simulink model "cooperative_observer"  (R2024b)
settings: Solver=VariableStepAuto  StartTime=0.0  StopTime=200  RelTol=1e-3
values from neighbouring files (symbols this model uses):
  A0 = A-B*K0    [Project.m]    (also in analyze_Ag_components.m = A - B*K0; analyze_Ao_components.m = A - B*K0; debug_simulink_integration.m = A - B*K0; local_observer_design.m = A - B*K0)
  Adj = ones(N, N) - eye(N)    [create_network_topology.m]    (also in debug_simulink_integration.m = zeros(N))
  B = [0; -9.9453]    [Project.m]    (also in debug_simulink_integration.m; find_hurwitz_F.m = c * eye(n); project_multiple_run.m; project_single_run.m)
  C = [708.27 0]    [Project.m]    (also in debug_simulink_integration.m; project_multiple_run.m; project_single_run.m)
  c = cmin * 2    [Project.m]    (also in project_multiple_run.m = cmin * c_weights(ic); project_single_run.m = cmin)
  D = zeros(1,2)    [Project.m]    (also in debug_simulink_integration.m = zeros(size(C,1), size(B,2)); project_multiple_run.m = zeros(1, 2); project_single_run.m = zeros(1, 2))
  F = P * C' * R^(-1)    [Project.m]    (also in find_hurwitz_F.m = reshape(F_opt, n, p); local_observer_design.m = place(A0', C', desired_poles)')
  G = zeros(N, N)    [create_network_topology.m]    (also in debug_simulink_integration.m = zeros(N))
  K = R^(-1) * B' *Pc    [Project.m]    (also in find_hurwitz_F.m = lqr(A, B, Q, R); project_multiple_run.m = R^(-1) * B' * Pc; project_single_run.m = R^(-1) * B' * Pc)
  L0 = place(A', C', [-10, -20])'    [Project.m]    (also in project_multiple_run.m = place(A0', C', [-10, -20])'; project_single_run.m = place(A0', C', [-10, -20])')
  x0_0 = [Amp 0]'    [Project.m]    (also in project_multiple_run.m = [Amp; 0]; project_single_run.m = [Amp; 0]; setup_ramp_parameters.m = [initial_value; slope; 0])
  x0_1 = [0 0]'    [Project.m]    (also in project_multiple_run.m = perturb(x0_0); project_single_run.m = perturb(x0_0))
  x0_2 = [0 0]'    [Project.m]    (also in project_multiple_run.m = perturb(x0_0); project_single_run.m = perturb(x0_0))
  x0_3 = [0 0]'    [Project.m]    (also in project_multiple_run.m = perturb(x0_0); project_single_run.m = perturb(x0_0))
  x0_4 = [0 0]'    [Project.m]    (also in project_multiple_run.m = perturb(x0_0); project_single_run.m = perturb(x0_0))
  x0_5 = [0 0]'    [Project.m]    (also in project_multiple_run.m = perturb(x0_0); project_single_run.m = perturb(x0_0))
  x0_6 = [0 0]'    [Project.m]    (also in project_multiple_run.m = perturb(x0_0); project_single_run.m = perturb(x0_0))
settings Model: Creator=fvero  LastModifiedBy=Ing. Dario Lupo

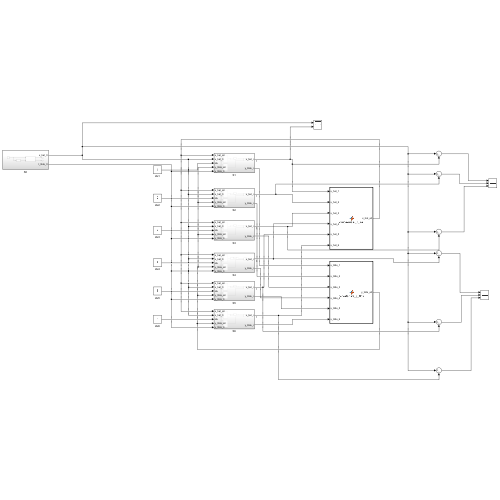
[thumbnail: Simulink's stored preview of the top-level diagram]
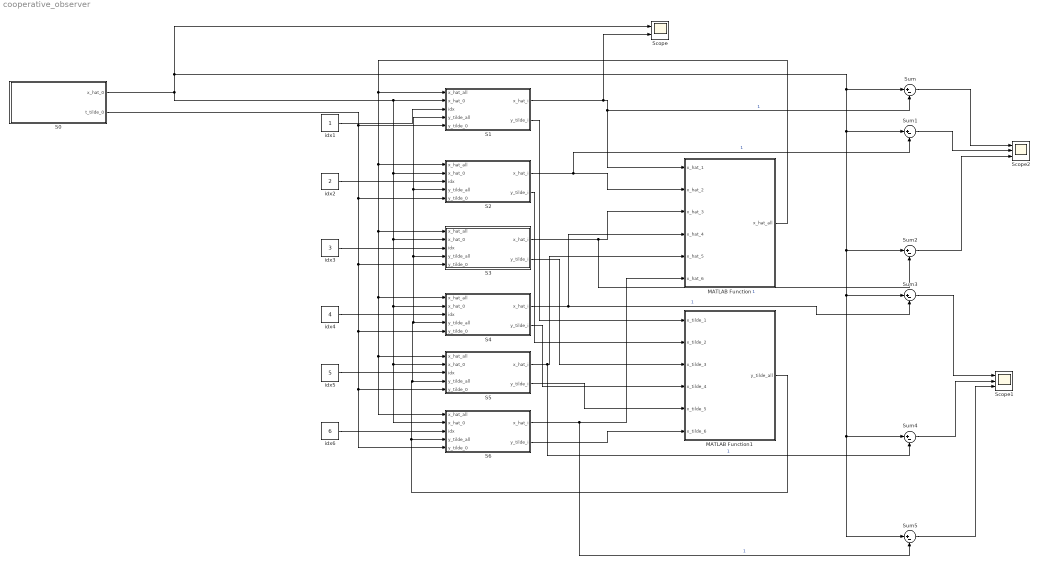
== system cooperative_observer ==
  MATLAB Function : MATLAB Function  TreatAsAtomicUnit=on
  MATLAB Function1 : MATLAB Function  TreatAsAtomicUnit=on
  S0 : Subsystem
  S1 : Subsystem
  S2 : Subsystem
  S3 : Subsystem
  S4 : Subsystem
  S5 : Subsystem
  S6 : Subsystem
  Scope : Scope  NumInputPorts=2
  Scope1 : Scope  NumInputPorts=3
  Scope2 : Scope  NumInputPorts=3
  Sum{,1..5} (6 alike) : Sum  Inputs=|+-
  idx1 : Constant
  idx2 : Constant  Value=2
  idx3 : Constant  Value=3
  idx4 : Constant  Value=4
  idx5 : Constant  Value=5
  idx6 : Constant  Value=6
  wires:
  MATLAB Function/1(x_hat_all) -> S6/1(x_hat_all), S5/1(x_hat_all), S4/1(x_hat_all), S3/1(x_hat_all), S2/1(x_hat_all), S1/1(x_hat_all)
  idx1/1 -> S1/3(idx)
  idx2/1 -> S2/3(idx)
  idx3/1 -> S3/3(idx)
  idx4/1 -> S4/3(idx)
  idx6/1 -> S6/3(idx)
  idx5/1 -> S5/3(idx)
  S0/1(x_hat_0) -> S6/2(x_hat_0), S5/2(x_hat_0), S4/2(x_hat_0), S3/2(x_hat_0), S2/2(x_hat_0), S1/2(x_hat_0), Scope/1, Sum4/1, Sum5/1, Sum3/1, Sum2/1, Sum1/1, Sum/1
  S1/1(x_hat_i) -> Scope/2, Sum/2, MATLAB Function/1(x_hat_1)  "1"
  S2/1(x_hat_i) -> Sum1/2, MATLAB Function/2(x_hat_2)  "1"
  S3/1(x_hat_i) -> Sum2/2, MATLAB Function/3(x_hat_3)  "1"
  S4/1(x_hat_i) -> Sum3/2, MATLAB Function/4(x_hat_4)  "1"
  S5/1(x_hat_i) -> Sum4/2, MATLAB Function/5(x_hat_5)  "1"
  S6/1(x_hat_i) -> Sum5/2, MATLAB Function/6(x_hat_6)  "1"
  S1/2(y_tilde_i) -> MATLAB Function1/1(x_tilde_1)
  S2/2(y_tilde_i) -> MATLAB Function1/2(x_tilde_2)
  S3/2(y_tilde_i) -> MATLAB Function1/3(x_tilde_3)
  S4/2(y_tilde_i) -> MATLAB Function1/4(x_tilde_4)
  S5/2(y_tilde_i) -> MATLAB Function1/5(x_tilde_5)
  S6/2(y_tilde_i) -> MATLAB Function1/6(x_tilde_6)
  MATLAB Function1/1(y_tilde_all) -> S2/4(y_tilde_all), S1/4(y_tilde_all), S3/4(y_tilde_all), S4/4(y_tilde_all), S5/4(y_tilde_all), S6/4(y_tilde_all)
  S0/2(t_tilde_0) -> S6/5(y_tilde_0), S5/5(y_tilde_0), S4/5(y_tilde_0), S3/5(y_tilde_0), S2/5(y_tilde_0), S1/5(y_tilde_0)
  Sum/1 -> Scope2/1
  Sum1/1 -> Scope2/2
  Sum2/1 -> Scope2/3
  Sum3/1 -> Scope1/1
  Sum4/1 -> Scope1/2
  Sum5/1 -> Scope1/3

== system cooperative_observer/S0 ==
  Constant : Constant  Value=0
  Leader Observer : Subsystem
  State-Space : StateSpace  A=A0  B=B  C=C  D=0  InitialCondition=x0_0
  x_hat_0 : Outport
  t_tilde_0 : Outport  Port=2
  wires:
  State-Space/1 -> Leader Observer/2(y)
  Constant/1 -> State-Space/1, Leader Observer/1(u)
  Leader Observer/1(x_hat_0) -> x_hat_0/1
  Leader Observer/2(t_tilde_0) -> t_tilde_0/1

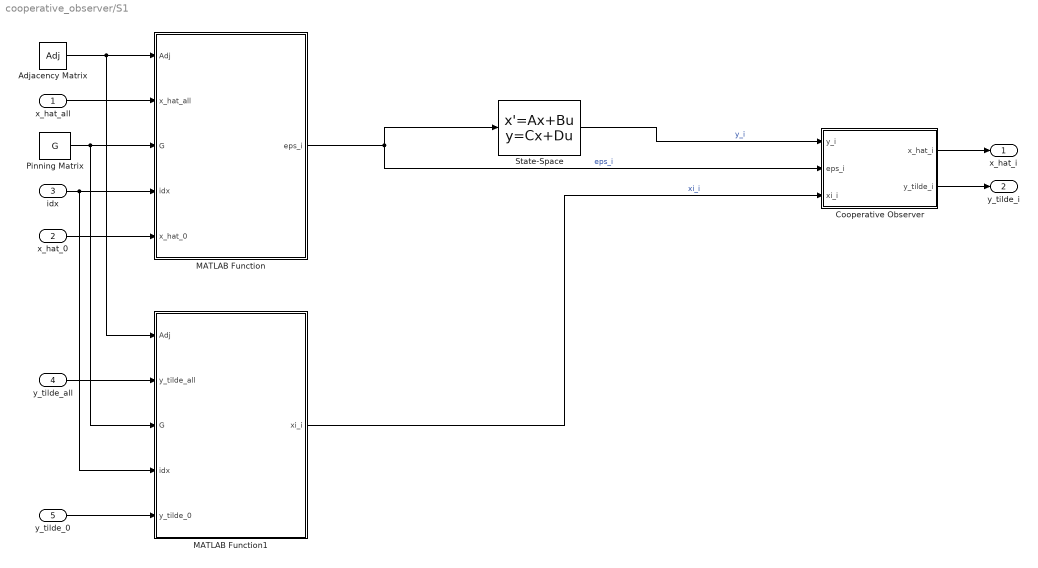
== system cooperative_observer/S1 ==
  x_hat_all : Inport
  x_hat_0 : Inport  Port=2
  idx : Inport  Port=3
  y_tilde_all : Inport  Port=4
  y_tilde_0 : Inport  Port=5
  "Adjacency Matrix " : Constant  Value=Adj
  Cooperative Observer : Subsystem
  MATLAB Function : MATLAB Function  TreatAsAtomicUnit=on
  MATLAB Function1 : MATLAB Function  TreatAsAtomicUnit=on
  Pinning Matrix : Constant  Value=G
  State-Space : StateSpace  A=A0  B=c*B*K  C=C  D=D  InitialCondition=x0_1
  x_hat_i : Outport
  y_tilde_i : Outport  Port=2
  wires:
  State-Space/1 -> Cooperative Observer/1(y_i)  "y_i"
  MATLAB Function/1(eps_i) -> State-Space/1, Cooperative Observer/2(eps_i)  "eps_i"
  x_hat_all/1 -> MATLAB Function/2(x_hat_all)
  x_hat_0/1 -> MATLAB Function/5(x_hat_0)
  Pinning Matrix/1 -> MATLAB Function1/3(G), MATLAB Function/3(G)
  "Adjacency Matrix "/1 -> MATLAB Function1/1(Adj), MATLAB Function/1(Adj)
  idx/1 -> MATLAB Function1/4(idx), MATLAB Function/4(idx)
  Cooperative Observer/1(x_hat_i) -> x_hat_i/1
  Cooperative Observer/2(y_tilde_i) -> y_tilde_i/1
  y_tilde_all/1 -> MATLAB Function1/2(y_tilde_all)
  y_tilde_0/1 -> MATLAB Function1/5(y_tilde_0)
  MATLAB Function1/1(xi_i) -> Cooperative Observer/3(xi_i)  "xi_i"

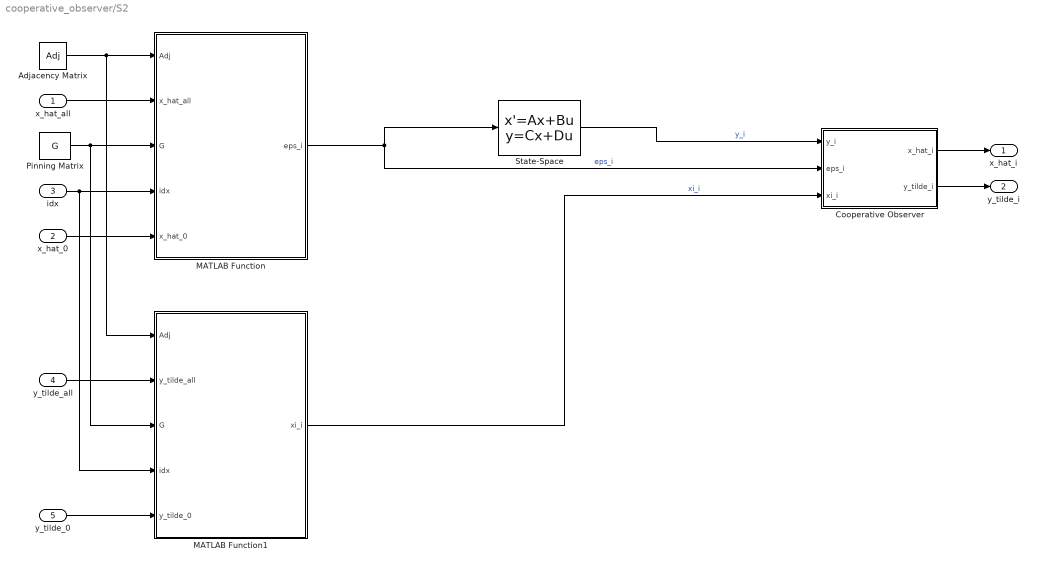
== system cooperative_observer/S2 ==
  x_hat_all : Inport
  x_hat_0 : Inport  Port=2
  idx : Inport  Port=3
  y_tilde_all : Inport  Port=4
  y_tilde_0 : Inport  Port=5
  "Adjacency Matrix " : Constant  Value=Adj
  Cooperative Observer : Subsystem
  MATLAB Function : MATLAB Function  TreatAsAtomicUnit=on
  MATLAB Function1 : MATLAB Function  TreatAsAtomicUnit=on
  Pinning Matrix : Constant  Value=G
  State-Space : StateSpace  A=A0  B=c*B*K  C=C  D=D  InitialCondition=x0_2
  x_hat_i : Outport
  y_tilde_i : Outport  Port=2
  wires:
  State-Space/1 -> Cooperative Observer/1(y_i)  "y_i"
  MATLAB Function/1(eps_i) -> State-Space/1, Cooperative Observer/2(eps_i)  "eps_i"
  x_hat_all/1 -> MATLAB Function/2(x_hat_all)
  x_hat_0/1 -> MATLAB Function/5(x_hat_0)
  Pinning Matrix/1 -> MATLAB Function1/3(G), MATLAB Function/3(G)
  "Adjacency Matrix "/1 -> MATLAB Function1/1(Adj), MATLAB Function/1(Adj)
  idx/1 -> MATLAB Function1/4(idx), MATLAB Function/4(idx)
  Cooperative Observer/1(x_hat_i) -> x_hat_i/1
  Cooperative Observer/2(y_tilde_i) -> y_tilde_i/1
  y_tilde_all/1 -> MATLAB Function1/2(y_tilde_all)
  y_tilde_0/1 -> MATLAB Function1/5(y_tilde_0)
  MATLAB Function1/1(xi_i) -> Cooperative Observer/3(xi_i)  "xi_i"

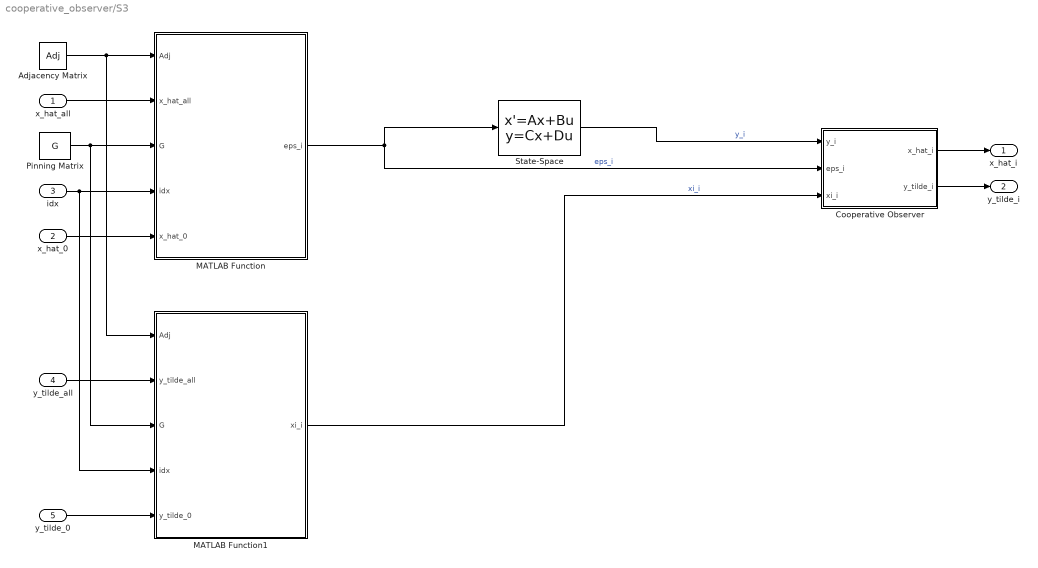
== system cooperative_observer/S3 ==
  x_hat_all : Inport
  x_hat_0 : Inport  Port=2
  idx : Inport  Port=3
  y_tilde_all : Inport  Port=4
  y_tilde_0 : Inport  Port=5
  "Adjacency Matrix " : Constant  Value=Adj
  Cooperative Observer : Subsystem
  MATLAB Function : MATLAB Function  TreatAsAtomicUnit=on
  MATLAB Function1 : MATLAB Function  TreatAsAtomicUnit=on
  Pinning Matrix : Constant  Value=G
  State-Space : StateSpace  A=A0  B=c*B*K  C=C  D=D  InitialCondition=x0_3
  x_hat_i : Outport
  y_tilde_i : Outport  Port=2
  wires:
  State-Space/1 -> Cooperative Observer/1(y_i)  "y_i"
  MATLAB Function/1(eps_i) -> State-Space/1, Cooperative Observer/2(eps_i)  "eps_i"
  x_hat_all/1 -> MATLAB Function/2(x_hat_all)
  x_hat_0/1 -> MATLAB Function/5(x_hat_0)
  Pinning Matrix/1 -> MATLAB Function1/3(G), MATLAB Function/3(G)
  "Adjacency Matrix "/1 -> MATLAB Function1/1(Adj), MATLAB Function/1(Adj)
  idx/1 -> MATLAB Function1/4(idx), MATLAB Function/4(idx)
  Cooperative Observer/1(x_hat_i) -> x_hat_i/1
  Cooperative Observer/2(y_tilde_i) -> y_tilde_i/1
  y_tilde_all/1 -> MATLAB Function1/2(y_tilde_all)
  y_tilde_0/1 -> MATLAB Function1/5(y_tilde_0)
  MATLAB Function1/1(xi_i) -> Cooperative Observer/3(xi_i)  "xi_i"

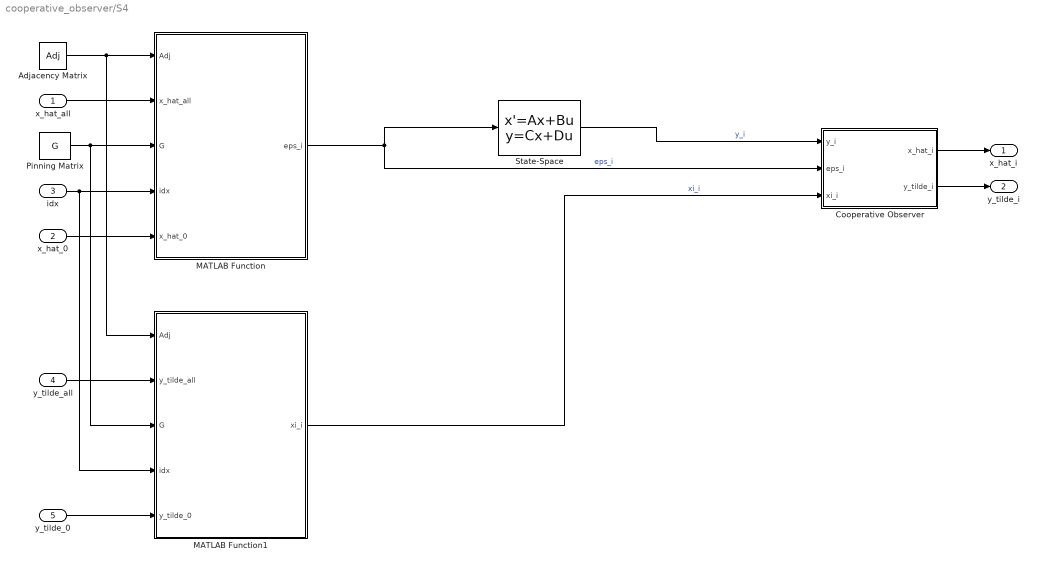
== system cooperative_observer/S4 ==
  x_hat_all : Inport
  x_hat_0 : Inport  Port=2
  idx : Inport  Port=3
  y_tilde_all : Inport  Port=4
  y_tilde_0 : Inport  Port=5
  "Adjacency Matrix " : Constant  Value=Adj
  Cooperative Observer : Subsystem
  MATLAB Function : MATLAB Function  TreatAsAtomicUnit=on
  MATLAB Function1 : MATLAB Function  TreatAsAtomicUnit=on
  Pinning Matrix : Constant  Value=G
  State-Space : StateSpace  A=A0  B=c*B*K  C=C  D=D  InitialCondition=x0_4
  x_hat_i : Outport
  y_tilde_i : Outport  Port=2
  wires:
  State-Space/1 -> Cooperative Observer/1(y_i)  "y_i"
  MATLAB Function/1(eps_i) -> State-Space/1, Cooperative Observer/2(eps_i)  "eps_i"
  x_hat_all/1 -> MATLAB Function/2(x_hat_all)
  x_hat_0/1 -> MATLAB Function/5(x_hat_0)
  Pinning Matrix/1 -> MATLAB Function1/3(G), MATLAB Function/3(G)
  "Adjacency Matrix "/1 -> MATLAB Function1/1(Adj), MATLAB Function/1(Adj)
  idx/1 -> MATLAB Function1/4(idx), MATLAB Function/4(idx)
  Cooperative Observer/1(x_hat_i) -> x_hat_i/1
  Cooperative Observer/2(y_tilde_i) -> y_tilde_i/1
  y_tilde_all/1 -> MATLAB Function1/2(y_tilde_all)
  y_tilde_0/1 -> MATLAB Function1/5(y_tilde_0)
  MATLAB Function1/1(xi_i) -> Cooperative Observer/3(xi_i)  "xi_i"

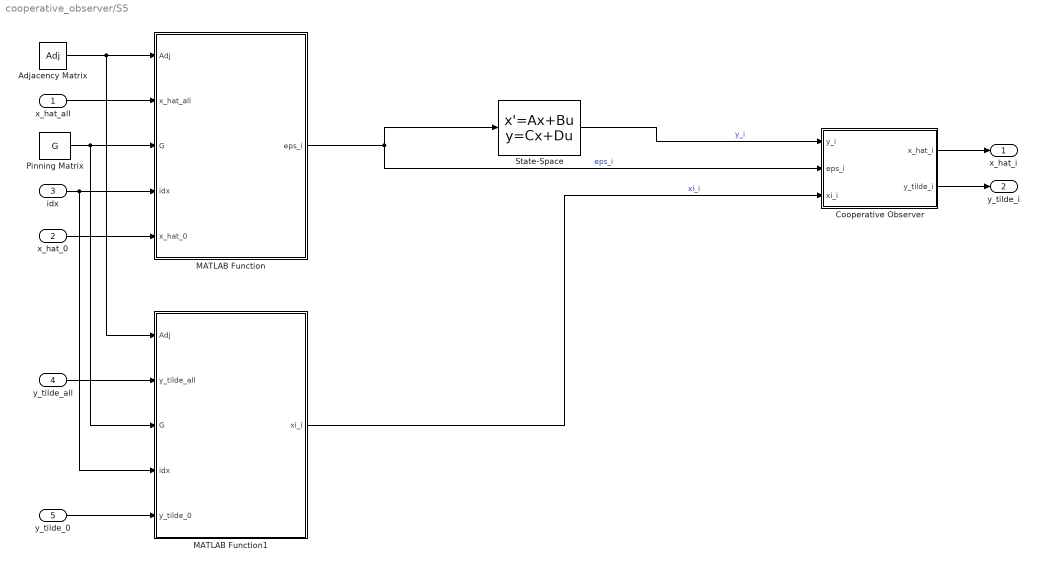
== system cooperative_observer/S5 ==
  x_hat_all : Inport
  x_hat_0 : Inport  Port=2
  idx : Inport  Port=3
  y_tilde_all : Inport  Port=4
  y_tilde_0 : Inport  Port=5
  "Adjacency Matrix " : Constant  Value=Adj
  Cooperative Observer : Subsystem
  MATLAB Function : MATLAB Function  TreatAsAtomicUnit=on
  MATLAB Function1 : MATLAB Function  TreatAsAtomicUnit=on
  Pinning Matrix : Constant  Value=G
  State-Space : StateSpace  A=A0  B=c*B*K  C=C  D=D  InitialCondition=x0_5
  x_hat_i : Outport
  y_tilde_i : Outport  Port=2
  wires:
  State-Space/1 -> Cooperative Observer/1(y_i)  "y_i"
  MATLAB Function/1(eps_i) -> State-Space/1, Cooperative Observer/2(eps_i)  "eps_i"
  x_hat_all/1 -> MATLAB Function/2(x_hat_all)
  x_hat_0/1 -> MATLAB Function/5(x_hat_0)
  Pinning Matrix/1 -> MATLAB Function1/3(G), MATLAB Function/3(G)
  "Adjacency Matrix "/1 -> MATLAB Function1/1(Adj), MATLAB Function/1(Adj)
  idx/1 -> MATLAB Function1/4(idx), MATLAB Function/4(idx)
  Cooperative Observer/1(x_hat_i) -> x_hat_i/1
  Cooperative Observer/2(y_tilde_i) -> y_tilde_i/1
  y_tilde_all/1 -> MATLAB Function1/2(y_tilde_all)
  y_tilde_0/1 -> MATLAB Function1/5(y_tilde_0)
  MATLAB Function1/1(xi_i) -> Cooperative Observer/3(xi_i)  "xi_i"

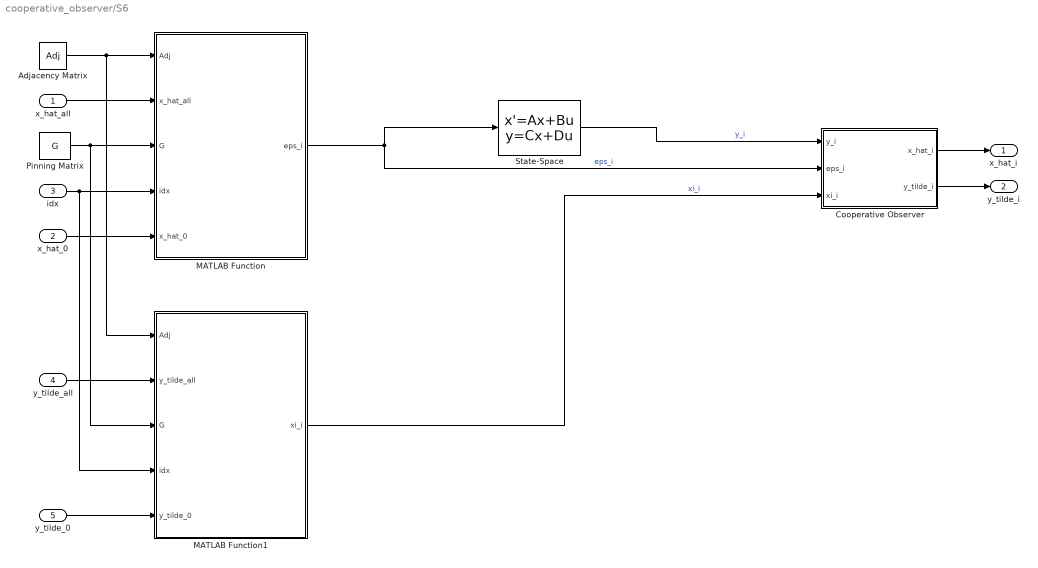
== system cooperative_observer/S6 ==
  x_hat_all : Inport
  x_hat_0 : Inport  Port=2
  idx : Inport  Port=3
  y_tilde_all : Inport  Port=4
  y_tilde_0 : Inport  Port=5
  "Adjacency Matrix " : Constant  Value=Adj
  Cooperative Observer : Subsystem
  MATLAB Function : MATLAB Function  TreatAsAtomicUnit=on
  MATLAB Function1 : MATLAB Function  TreatAsAtomicUnit=on
  Pinning Matrix : Constant  Value=G
  State-Space : StateSpace  A=A0  B=c*B*K  C=C  D=D  InitialCondition=x0_6
  x_hat_i : Outport
  y_tilde_i : Outport  Port=2
  wires:
  State-Space/1 -> Cooperative Observer/1(y_i)  "y_i"
  MATLAB Function/1(eps_i) -> State-Space/1, Cooperative Observer/2(eps_i)  "eps_i"
  x_hat_all/1 -> MATLAB Function/2(x_hat_all)
  x_hat_0/1 -> MATLAB Function/5(x_hat_0)
  Pinning Matrix/1 -> MATLAB Function1/3(G), MATLAB Function/3(G)
  "Adjacency Matrix "/1 -> MATLAB Function1/1(Adj), MATLAB Function/1(Adj)
  idx/1 -> MATLAB Function1/4(idx), MATLAB Function/4(idx)
  Cooperative Observer/1(x_hat_i) -> x_hat_i/1
  Cooperative Observer/2(y_tilde_i) -> y_tilde_i/1
  y_tilde_all/1 -> MATLAB Function1/2(y_tilde_all)
  y_tilde_0/1 -> MATLAB Function1/5(y_tilde_0)
  MATLAB Function1/1(xi_i) -> Cooperative Observer/3(xi_i)  "xi_i"

== system cooperative_observer/S0/Leader Observer ==
  u : Inport
  y : Inport  Port=2
  Add : Sum  Inputs=+++
  Add1 : Sum  Inputs=+-
  Gain : Gain  Gain=B  Multiplication=Matrix(K*u)
  Gain1 : Gain  Gain=A0  Multiplication=Matrix(K*u)
  Gain2 : Gain  Gain=C  Multiplication=Matrix(K*u)
  Gain3 : Gain  Gain=c*L0  Multiplication=Matrix(K*u)
  Integrator : Integrator  InitialCondition=x0_0
  x_hat_0 : Outport
  t_tilde_0 : Outport  Port=2
  wires:
  u/1 -> Gain/1
  Gain/1 -> Add/1
  Add/1 -> Integrator/1  "x_hat_dot"
  y/1 -> Add1/1
  Integrator/1 -> x_hat_0/1, Gain2/1, Gain1/1  "x_hat"
  Gain2/1 -> Add1/2  "y_hat"
  Gain1/1 -> Add/3
  Add1/1 -> t_tilde_0/1, Gain3/1  "y_tilde"
  Gain3/1 -> Add/2

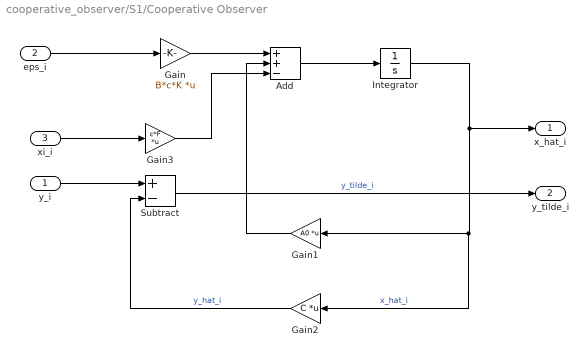
== system cooperative_observer/S1/Cooperative Observer ==
  y_i : Inport
  eps_i : Inport  Port=2
  xi_i : Inport  Port=3
  Add : Sum  Inputs=++-
  Gain : Gain  Gain=B*c*K  Multiplication=Matrix(K*u)
  Gain1 : Gain  Gain=A0  Multiplication=Matrix(K*u)
  Gain2 : Gain  Gain=C  Multiplication=Matrix(K*u)
  Gain3 : Gain  Gain=c*F  Multiplication=Matrix(K*u)
  Integrator : Integrator  InitialCondition=x0_1
  Subtract : Sum  Inputs=+-
  x_hat_i : Outport
  y_tilde_i : Outport  Port=2
  wires:
  eps_i/1 -> Gain/1
  Integrator/1 -> Gain2/1, Gain1/1, x_hat_i/1  "x_hat_i"
  y_i/1 -> Subtract/1
  Gain2/1 -> Subtract/2  "y_hat_i"
  Subtract/1 -> y_tilde_i/1  "y_tilde_i"
  Gain/1 -> Add/1
  Gain3/1 -> Add/3
  Gain1/1 -> Add/2
  Add/1 -> Integrator/1
  xi_i/1 -> Gain3/1

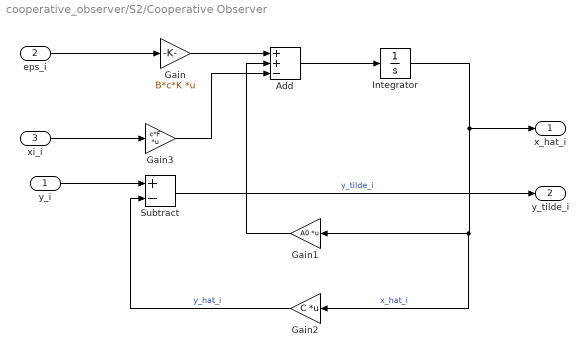
== system cooperative_observer/S2/Cooperative Observer ==
  y_i : Inport
  eps_i : Inport  Port=2
  xi_i : Inport  Port=3
  Add : Sum  Inputs=++-
  Gain : Gain  Gain=B*c*K  Multiplication=Matrix(K*u)
  Gain1 : Gain  Gain=A0  Multiplication=Matrix(K*u)
  Gain2 : Gain  Gain=C  Multiplication=Matrix(K*u)
  Gain3 : Gain  Gain=c*F  Multiplication=Matrix(K*u)
  Integrator : Integrator  InitialCondition=x0_2
  Subtract : Sum  Inputs=+-
  x_hat_i : Outport
  y_tilde_i : Outport  Port=2
  wires:
  eps_i/1 -> Gain/1
  Integrator/1 -> Gain2/1, Gain1/1, x_hat_i/1  "x_hat_i"
  y_i/1 -> Subtract/1
  Gain2/1 -> Subtract/2  "y_hat_i"
  Subtract/1 -> y_tilde_i/1  "y_tilde_i"
  Gain/1 -> Add/1
  Gain3/1 -> Add/3
  Gain1/1 -> Add/2
  Add/1 -> Integrator/1
  xi_i/1 -> Gain3/1

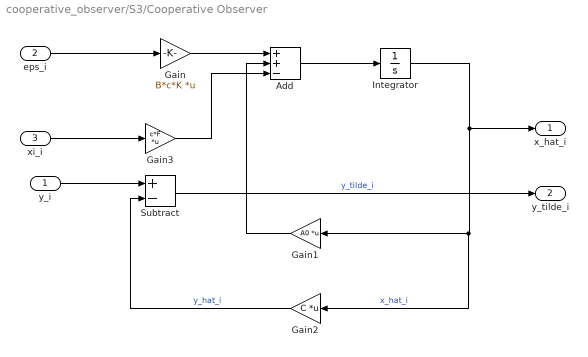
== system cooperative_observer/S3/Cooperative Observer ==
  y_i : Inport
  eps_i : Inport  Port=2
  xi_i : Inport  Port=3
  Add : Sum  Inputs=++-
  Gain : Gain  Gain=B*c*K  Multiplication=Matrix(K*u)
  Gain1 : Gain  Gain=A0  Multiplication=Matrix(K*u)
  Gain2 : Gain  Gain=C  Multiplication=Matrix(K*u)
  Gain3 : Gain  Gain=c*F  Multiplication=Matrix(K*u)
  Integrator : Integrator  InitialCondition=x0_3
  Subtract : Sum  Inputs=+-
  x_hat_i : Outport
  y_tilde_i : Outport  Port=2
  wires:
  eps_i/1 -> Gain/1
  Integrator/1 -> Gain2/1, Gain1/1, x_hat_i/1  "x_hat_i"
  y_i/1 -> Subtract/1
  Gain2/1 -> Subtract/2  "y_hat_i"
  Subtract/1 -> y_tilde_i/1  "y_tilde_i"
  Gain/1 -> Add/1
  Gain3/1 -> Add/3
  Gain1/1 -> Add/2
  Add/1 -> Integrator/1
  xi_i/1 -> Gain3/1

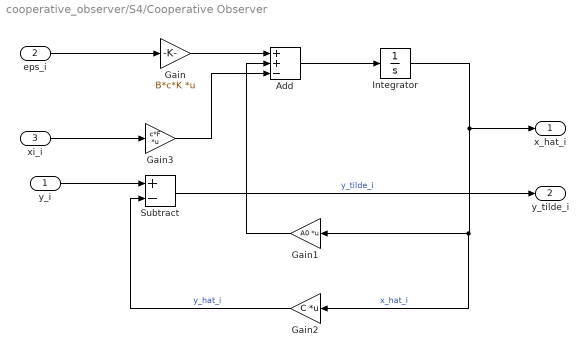
== system cooperative_observer/S4/Cooperative Observer ==
  y_i : Inport
  eps_i : Inport  Port=2
  xi_i : Inport  Port=3
  Add : Sum  Inputs=++-
  Gain : Gain  Gain=B*c*K  Multiplication=Matrix(K*u)
  Gain1 : Gain  Gain=A0  Multiplication=Matrix(K*u)
  Gain2 : Gain  Gain=C  Multiplication=Matrix(K*u)
  Gain3 : Gain  Gain=c*F  Multiplication=Matrix(K*u)
  Integrator : Integrator  InitialCondition=x0_4
  Subtract : Sum  Inputs=+-
  x_hat_i : Outport
  y_tilde_i : Outport  Port=2
  wires:
  eps_i/1 -> Gain/1
  Integrator/1 -> Gain2/1, Gain1/1, x_hat_i/1  "x_hat_i"
  y_i/1 -> Subtract/1
  Gain2/1 -> Subtract/2  "y_hat_i"
  Subtract/1 -> y_tilde_i/1  "y_tilde_i"
  Gain/1 -> Add/1
  Gain3/1 -> Add/3
  Gain1/1 -> Add/2
  Add/1 -> Integrator/1
  xi_i/1 -> Gain3/1

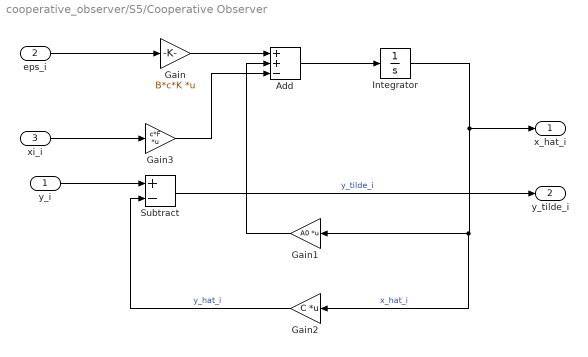
== system cooperative_observer/S5/Cooperative Observer ==
  y_i : Inport
  eps_i : Inport  Port=2
  xi_i : Inport  Port=3
  Add : Sum  Inputs=++-
  Gain : Gain  Gain=B*c*K  Multiplication=Matrix(K*u)
  Gain1 : Gain  Gain=A0  Multiplication=Matrix(K*u)
  Gain2 : Gain  Gain=C  Multiplication=Matrix(K*u)
  Gain3 : Gain  Gain=c*F  Multiplication=Matrix(K*u)
  Integrator : Integrator  InitialCondition=x0_5
  Subtract : Sum  Inputs=+-
  x_hat_i : Outport
  y_tilde_i : Outport  Port=2
  wires:
  eps_i/1 -> Gain/1
  Integrator/1 -> Gain2/1, Gain1/1, x_hat_i/1  "x_hat_i"
  y_i/1 -> Subtract/1
  Gain2/1 -> Subtract/2  "y_hat_i"
  Subtract/1 -> y_tilde_i/1  "y_tilde_i"
  Gain/1 -> Add/1
  Gain3/1 -> Add/3
  Gain1/1 -> Add/2
  Add/1 -> Integrator/1
  xi_i/1 -> Gain3/1

== system cooperative_observer/S6/Cooperative Observer ==
  y_i : Inport
  eps_i : Inport  Port=2
  xi_i : Inport  Port=3
  Add : Sum  Inputs=++-
  Gain : Gain  Gain=B*c*K  Multiplication=Matrix(K*u)
  Gain1 : Gain  Gain=A0  Multiplication=Matrix(K*u)
  Gain2 : Gain  Gain=C  Multiplication=Matrix(K*u)
  Gain3 : Gain  Gain=c*F  Multiplication=Matrix(K*u)
  Integrator : Integrator  InitialCondition=x0_6
  Subtract : Sum  Inputs=+-
  x_hat_i : Outport
  y_tilde_i : Outport  Port=2
  wires:
  eps_i/1 -> Gain/1
  Integrator/1 -> Gain2/1, Gain1/1, x_hat_i/1  "x_hat_i"
  y_i/1 -> Subtract/1
  Gain2/1 -> Subtract/2  "y_hat_i"
  Subtract/1 -> y_tilde_i/1  "y_tilde_i"
  Gain/1 -> Add/1
  Gain3/1 -> Add/3
  Gain1/1 -> Add/2
  Add/1 -> Integrator/1
  xi_i/1 -> Gain3/1

== matlab function cooperative_observer/S4/MATLAB Function1 ==
  data: Adj input; xi_i output; y_tilde_all input; G input; idx input; y_tilde_0 input
function xi_i = compute_xi(Adj, y_tilde_all, G, idx, y_tilde_0)

Adj_i = Adj(idx, :);
g_i = G(idx, idx);

y_tilde_i = y_tilde_all(idx); 

diff = g_i * (y_tilde_0 - y_tilde_i); 

xi_i = 0; 

for j = 1:6
    xi_i = xi_i + Adj_i(j)*(y_tilde_all(j) - y_tilde_i) + diff; 
end 

end

== matlab function cooperative_observer/S5/MATLAB Function ==
  data: Adj input; eps_i output; x_hat_all input; G input; idx input; x_hat_0 input
function eps_i = compute_eps(Adj, x_hat_all, G, idx, x_hat_0)

Adj_i = Adj(idx, :);
g_i = G(idx, idx);

x_hat_i = x_hat_all(idx, :)'; %2*1

diff = g_i * (x_hat_0 - x_hat_i); 

eps_i = zeros(size(x_hat_i)); 

for j = 1:6
    eps_i = eps_i + Adj_i(j)*(x_hat_all(j,:)' - x_hat_i) + diff; 
end 

end

== matlab function cooperative_observer/MATLAB Function1 ==
  data: x_tilde_1 input; y_tilde_all output; x_tilde_2 input; x_tilde_3 input; x_tilde_4 input; x_tilde_5 input; x_tilde_6 input
function y_tilde_all = concatenate_y_tilde(x_tilde_1, x_tilde_2, x_tilde_3, x_tilde_4, x_tilde_5, x_tilde_6)

y_tilde_all = [x_tilde_1 x_tilde_2 x_tilde_3 x_tilde_4 x_tilde_5 x_tilde_6];

end

== matlab function cooperative_observer/S5/MATLAB Function1 ==
  data: Adj input; xi_i output; y_tilde_all input; G input; idx input; y_tilde_0 input
function xi_i = compute_xi(Adj, y_tilde_all, G, idx, y_tilde_0)

Adj_i = Adj(idx, :);
g_i = G(idx, idx);

y_tilde_i = y_tilde_all(idx); 

diff = g_i * (y_tilde_0 - y_tilde_i); 

xi_i = 0; 

for j = 1:6
    xi_i = xi_i + Adj_i(j)*(y_tilde_all(j) - y_tilde_i) + diff; 
end 

end

== matlab function cooperative_observer/S6/MATLAB Function ==
  data: Adj input; eps_i output; x_hat_all input; G input; idx input; x_hat_0 input
function eps_i = compute_eps(Adj, x_hat_all, G, idx, x_hat_0)

Adj_i = Adj(idx, :);
g_i = G(idx, idx);

x_hat_i = x_hat_all(idx, :)'; %2*1

diff = g_i * (x_hat_0 - x_hat_i); 

eps_i = zeros(size(x_hat_i)); 

for j = 1:6
    eps_i = eps_i + Adj_i(j)*(x_hat_all(j,:)' - x_hat_i) + diff; 
end 

end

== matlab function cooperative_observer/S6/MATLAB Function1 ==
  data: Adj input; xi_i output; y_tilde_all input; G input; idx input; y_tilde_0 input
function xi_i = compute_xi(Adj, y_tilde_all, G, idx, y_tilde_0)

Adj_i = Adj(idx, :);
g_i = G(idx, idx);

y_tilde_i = y_tilde_all(idx); 

diff = g_i * (y_tilde_0 - y_tilde_i); 

xi_i = 0; 

for j = 1:6
    xi_i = xi_i + Adj_i(j)*(y_tilde_all(j) - y_tilde_i) + diff; 
end 

end

== matlab function cooperative_observer/MATLAB Function ==
  data: x_hat_1 input; x_hat_all output; x_hat_2 input; x_hat_3 input; x_hat_4 input; x_hat_5 input; x_hat_6 input
function x_hat_all = concatenate_x_hat(x_hat_1, x_hat_2, x_hat_3, x_hat_4, x_hat_5, x_hat_6)

x_hat_all = [x_hat_1'; x_hat_2'; x_hat_3'; x_hat_4'; x_hat_5'; x_hat_6'];

end

== matlab function cooperative_observer/S1/MATLAB Function ==
  data: Adj input; eps_i output; x_hat_all input; G input; idx input; x_hat_0 input
function eps_i = compute_eps(Adj, x_hat_all, G, idx, x_hat_0)

Adj_i = Adj(idx, :);
g_i = G(idx, idx);

x_hat_i = x_hat_all(idx, :)'; %2*1

diff = g_i * (x_hat_0 - x_hat_i); 

eps_i = zeros(size(x_hat_i)); 

for j = 1:6
    eps_i = eps_i + Adj_i(j)*(x_hat_all(j,:)' - x_hat_i) + diff; 
end 

end

== matlab function cooperative_observer/S1/MATLAB Function1 ==
  data: Adj input; xi_i output; y_tilde_all input; G input; idx input; y_tilde_0 input
function xi_i = compute_xi(Adj, y_tilde_all, G, idx, y_tilde_0)

Adj_i = Adj(idx, :);
g_i = G(idx, idx);

y_tilde_i = y_tilde_all(idx); 

diff = g_i * (y_tilde_0 - y_tilde_i); 

xi_i = 0; 

for j = 1:6
    xi_i = xi_i + Adj_i(j)*(y_tilde_all(j) - y_tilde_i) + diff; 
end 

end

== matlab function cooperative_observer/S2/MATLAB Function ==
  data: Adj input; eps_i output; x_hat_all input; G input; idx input; x_hat_0 input
function eps_i = compute_eps(Adj, x_hat_all, G, idx, x_hat_0)

Adj_i = Adj(idx, :);
g_i = G(idx, idx);

x_hat_i = x_hat_all(idx, :)'; %2*1

diff = g_i * (x_hat_0 - x_hat_i); 

eps_i = zeros(size(x_hat_i)); 

for j = 1:6
    eps_i = eps_i + Adj_i(j)*(x_hat_all(j,:)' - x_hat_i) + diff; 
end 

end

== matlab function cooperative_observer/S2/MATLAB Function1 ==
  data: Adj input; xi_i output; y_tilde_all input; G input; idx input; y_tilde_0 input
function xi_i = compute_xi(Adj, y_tilde_all, G, idx, y_tilde_0)

Adj_i = Adj(idx, :);
g_i = G(idx, idx);

y_tilde_i = y_tilde_all(idx); 

diff = g_i * (y_tilde_0 - y_tilde_i); 

xi_i = 0; 

for j = 1:6
    xi_i = xi_i + Adj_i(j)*(y_tilde_all(j) - y_tilde_i) + diff; 
end 

end

== matlab function cooperative_observer/S3/MATLAB Function ==
  data: Adj input; eps_i output; x_hat_all input; G input; idx input; x_hat_0 input
function eps_i = compute_eps(Adj, x_hat_all, G, idx, x_hat_0)

Adj_i = Adj(idx, :);
g_i = G(idx, idx);

x_hat_i = x_hat_all(idx, :)'; %2*1

diff = g_i * (x_hat_0 - x_hat_i); 

eps_i = zeros(size(x_hat_i)); 

for j = 1:6
    eps_i = eps_i + Adj_i(j)*(x_hat_all(j,:)' - x_hat_i) + diff; 
end 

end

== matlab function cooperative_observer/S3/MATLAB Function1 ==
  data: Adj input; xi_i output; y_tilde_all input; G input; idx input; y_tilde_0 input
function xi_i = compute_xi(Adj, y_tilde_all, G, idx, y_tilde_0)

Adj_i = Adj(idx, :);
g_i = G(idx, idx);

y_tilde_i = y_tilde_all(idx); 

diff = g_i * (y_tilde_0 - y_tilde_i); 

xi_i = 0; 

for j = 1:6
    xi_i = xi_i + Adj_i(j)*(y_tilde_all(j) - y_tilde_i) + diff; 
end 

end

== matlab function cooperative_observer/S4/MATLAB Function ==
  data: Adj input; eps_i output; x_hat_all input; G input; idx input; x_hat_0 input
function eps_i = compute_eps(Adj, x_hat_all, G, idx, x_hat_0)

Adj_i = Adj(idx, :);
g_i = G(idx, idx);

x_hat_i = x_hat_all(idx, :)'; %2*1

diff = g_i * (x_hat_0 - x_hat_i); 

eps_i = zeros(size(x_hat_i)); 

for j = 1:6
    eps_i = eps_i + Adj_i(j)*(x_hat_all(j,:)' - x_hat_i) + diff; 
end 

end
